simulink library "MIL_Test"  (Simulink 6.6)
undefined symbols (not defined in the file or in its folder): getdatatypespecs, slcm, StepSize
libraries: simulink x71, MIL_Test x6
(part 1 of 8)
settings Model: Creator=Justyna  LastModifiedBy=Justyna

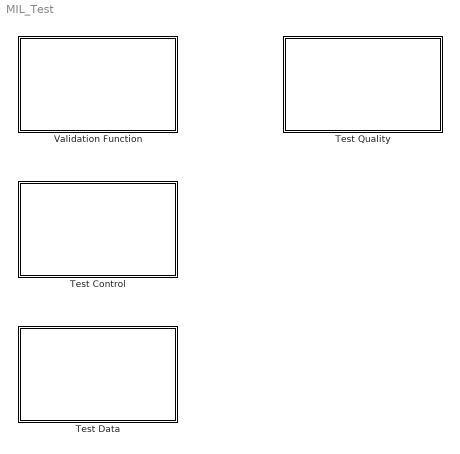
== system MIL_Test ==
  Test Control : Subsystem
  Test Data : Subsystem
  Test Quality : Subsystem
  Validation Function : Subsystem

== system MIL_Test/Test Control ==
  Test Control : Subsystem
  Test Control Architecture : Subsystem

== system MIL_Test/Test Data ==
  Feature generation : Subsystem
  Signal comparison : Subsystem
  Test Data Architecture : Subsystem

== system MIL_Test/Test Quality ==
  VFs Activation  Coverage : Subsystem  mask{req=9, So=on}
      mask prompts: req "Number of Evaluated Scenarios within Requirements"; So "Adjust to the present Eva Results"
      mask StyleString: popup(1|2|3|4|5|6|7|8|9|10|11|12|13|14|15|16|17|18|19|20),checkbox
      mask CallbackString: |Requirements_Coverage_callback(gcb,-1)

== system MIL_Test/Validation Function ==
  Assertions : MIL_Test/Validation Function/TODO/Assertions  SystemSampleTime=-1
  Feature extraction : Subsystem
  Preconditions : MIL_Test/Validation Function/TODO/Preconditions  SystemSampleTime=-1
  Signal comparison : Subsystem
  TODO : Subsystem
  Test Evaluation Architecture : Subsystem

== system MIL_Test/Test Control/Test Control ==

== system MIL_Test/Test Control/Test Control Architecture ==
  Connection Helpers : Subsystem
  Test Control  depending on Verdict : Subsystem  Orientation=left
  Test Control Conditions : Subsystem
  "independent  Test Control " : Stateflow chart  Orientation=left

== system MIL_Test/Test Data/Feature generation ==
  Generate  feature variants : Subsystem
  Generate  limited decrease : Subsystem  mask(Feature generation){X0=0.5, XF=0}
      mask prompts: X0 "Initial output:"; XF "Final output:"
      mask help: Output a decreasing ramp signal limited from bottom and top, starting at the specified time.
      mask Display:
      | plot([1:10],[4,4,4,4,4,1,1,1,1,1])
      | plot([1:10],[4,4,4,1,1,1,1,1,1,1])
      | plot([1:10],[4,1,1,1,1,1,1,1,1,1])
      | plot([1:10],[4,4,4,4,4,1,1,1,1,1])
      | plot([1:10],[4,4,4,4,4,4,4,1,1,1])
      | plot([1:10],[4,4,4,4,4,4,4,4,4,1])
      | plot([1:10],[4,4,4,4,4,4,4,4,4,4])
      | color('white');
      | plot([1:10],[1,1,1,1,1,1,1,1,1,1])
      | color('black');
      | plot([1,1.5],[1,1])
      | plot([2.5,3.5],[1,1])
      | plot([4.5,5.5],[1,1])
      | plot([6.5,7.5],[1,1])
      | plot([8.5,9.5],[1,1])
      | color('white');
      | plot([1,1.5],[4,4])
      | plot([2.5,3.5],[4,4])
      | plot([4.5,5.5],[4,4])
      | plot([6.5,7.5],[4,4])
      | plot([8.5,9.5],[4,4])
  Generate  limited decrease  with slope : Subsystem  mask(Feature generation){slope=-0.5, start=0, X0=100, XF=10, VectorParams1D=on}
      mask prompts: start "Start time:"; X0 "Initial output:"; XF "Final output:"; VectorParams1D "Interpret vector parameters as 1-D"
      mask help: Output a decreasing ramp signal limited from bottom and top, starting at the specified time.
      mask init:
      | blkName = gcb;
      | set_param([blkName '/Constant'], 'VectorParams1D',VectorParams1D);
      | set_param([blkName '/Constant1'], 'VectorParams1D',VectorParams1D);
      | set_param([blkName '/Step'], 'VectorParams1D',VectorParams1D);
      mask Display:
      | plot([1:10],[4,4,4,4,4,1,1,1,1,1])
      | plot([1:10],[4,4,4,4,4,4,4,4,4,4])
      | color('white');
      | plot([1:10],[1,1,1,1,1,1,1,1,1,1])
      | color('black');
      | plot([1,1.5],[1,1])
      | plot([2.5,3.5],[1,1])
      | plot([4.5,5.5],[1,1])
      | plot([6.5,7.5],[1,1])
      | plot([8.5,9.5],[1,1])
      | color('white');
      | plot([1,1.5],[4,4])
      | plot([2.5,3.5],[4,4])
      | plot([4.5,5.5],[4,4])
      | plot([6.5,7.5],[4,4])
      | plot([8.5,9.5],[4,4])
  Generate  limited increase : Subsystem  mask(Feature generation){X0=5, XF=14.5}
      mask prompts: X0 "Initial output:"; XF "Final output:"
      mask help: Output a ramp signal limited from bottom and top, starting at the specified time.
      mask Display:
      | plot([1:10],[1,1,1,1,1,4,4,4,4,4])
      | plot([1:10],[1,4,4,4,4,4,4,4,4,4])
      | plot([1:10],[1,1,1,4,4,4,4,4,4,4])
      | plot([1:10],[1,1,1,1,1,4,4,4,4,4])
      | plot([1:10],[1,1,1,1,1,1,1,4,4,4])
      | plot([1:10],[1,1,1,1,1,1,1,1,1,4])
      | plot([5:10],[1,1,1,1,1,1])
      | color('white');
      | plot([1:10],[4,4,4,4,4,4,4,4,4,4])
      | color('white');
      | plot([1,1.5],[1,1])
      | plot([2.5,3.5],[1,1])
      | plot([4.5,5.5],[1,1])
      | plot([6.5,7.5],[1,1])
      | plot([8.5,9.5],[1,1])
      | color('black');
      | plot([1,1.5],[4,4])
      | plot([2.5,3.5],[4,4])
      | plot([4.5,5.5],[4,4])
      | plot([6.5,7.5],[4,4])
      | plot([8.5,9.5],[4,4])
  Generate  limited increase  with slope : Subsystem  mask(Feature generation){slope=3.5, start=0, X0=10, XF=50, VectorParams1D=on}
      mask prompts: start "Start time:"; X0 "Initial output:"; XF "Final output:"; VectorParams1D "Interpret vector parameters as 1-D"
      mask help: Output a ramp signal limited from bottom and top, starting at the specified time.
      mask init: same as MIL_Test/Test Data/Feature generation/Generate  limited decrease  with slope
      mask Display:
      | plot([1:10],[1,1,1,1,1,4,4,4,4,4])
      | plot([5:10],[1,1,1,1,1,1])
      | color('white');
      | plot([1:10],[4,4,4,4,4,4,4,4,4,4])
      | color('white');
      | plot([1,1.5],[1,1])
      | plot([2.5,3.5],[1,1])
      | plot([4.5,5.5],[1,1])
      | plot([6.5,7.5],[1,1])
      | plot([8.5,9.5],[1,1])
      | color('black');
      | plot([1,1.5],[4,4])
      | plot([2.5,3.5],[4,4])
      | plot([4.5,5.5],[4,4])
      | plot([6.5,7.5],[4,4])
      | plot([8.5,9.5],[4,4])
  "Generate  local maximum  @ given time " : Subsystem  TreatAsAtomicUnit=on  mask(Feature generation){maxt=8, X0=10, XF=100}
      mask prompts: maxt "Time of Max:"; X0 "Lower Limit:"; XF "Upper Limit:"
      mask help: Generate local maximum
      mask Display:
      | plot([1:9],[1,1,1,1,4,1,1,1,1])
      | text(6,3,'@time')
  Generate  local maximum  with given slope : Subsystem  TreatAsAtomicUnit=on  mask(Feature generation){slope=7, start=5, maxt=8, X0=10, XF=100}
      mask prompts: start "Start Time of Feature:"; maxt "Time of Max:"; X0 "Lower Limit:"; XF "Upper Limit:"
      mask help: Generate local maximum
      mask Display:
      | plot([1:9],[1,1,1,1,4,1,1,1,1])
      | text(2,2,'slope')
      | text(6,3,'@time')
  Generate  local maximum = maxvalue  @ given time : Subsystem  TreatAsAtomicUnit=on  mask(Feature generation){maxv=50, maxt=5, X0=10}
      mask prompts: maxv "Value of Max:"; maxt "Time of Max:"; X0 "Lower Limit:"
      mask help: Generate local maximum = specified value
      mask Display:
      | plot([1:7],[1,1,4,1,1,1,1])
      | text(3.8,3.5,'max value')
      | text(4.1,2.5,'@time')
  Generate any step response  characteristics : Subsystem  mask(Feature generation){Param=0}
      mask prompts: Param "Mask Parameter 1:"
      mask help: Generate any step response characteristics
      mask Display:
      | plot([1:23],[-1,-1,-1,-1,0.3,1,1.5,1.7,1.5,0.7,0.4,0.6,1.1,1,0.6,0.7,0.7,0.7,0.7,0.7,0.7,0.7,0.7])
      | patch(0.17+[0.7 0.6 0.6 0.65 0.6 0.6 0.7],-0.043+[0.7 0.63 0.64 0.7 0.76 0.77 0.7],[0 0 0]);
  Generate complete step : Subsystem  mask(Complete step detection){Param=0}
      mask prompts: Param "Mask Parameter 1:"
      mask Display: plot([1,2,3,4,4.0001,6,7,7.0001,9,10],[1,1,1,1,4,4,4,2,2,2])
  Generate constant : Constant  Value=0  OutDataTypeMode=boolean
  Generate linear relation : Subsystem  mask(Feature generation){c=}
      mask prompts: c "Slope - c parameter:"
      mask help: Linear function y=cu
      mask Display:
      | plot([0:10],[0,1:10])
      | text(1,6.5,'y = c*u')
  Generate min to date : Subsystem  mask(Feature generation){low=-3, up=10}
      mask prompts: low "Min - Lower limit:"; up "Max - Upper limit:"
      mask help: Generate any characteristics
      mask Display:
      | port_label('output',1,'Min to date');
      | patch(0.05+[0.25 0.25 0.8 0.8 0.26 0.26],[0.95 0.65 0.65 0.66 0.66 0.95],[0 0 0]);
      | patch(0.033+[0.27 0.22 0.23 0.27 0.31 0.32 0.27],0.02+[0.95 0.85 0.85 0.89 0.85 0.85 0.95],[0 0 0]);
      | patch(0.27+[0.7 0.6 0.6 0.65 0.6 0.6 0.7],-0.043+[0.7 0.63 0.64 0.7 0.76 0.77 0.7],[0 0 0]);
      | patch(0.05+[0.25 0.25 0.25 0.5 0.26 0.26],0.05+[0.65 0.65 0.65 0.66 0.66 0.95],[0 0 0]);
  Generate peaks : Subsystem  TreatAsAtomicUnit=on  mask(Feature generation){Sens=0.910, freq=1}
      mask prompts: Sens "Peak value:"; freq "Peaks frequency:"
      mask help: Generate a peak in a signal. The peak might be positive or negative. The user-defined parameter define the minimal peak size and frequency of peak occurence.
      mask CallbackString:
      | if str2double(get_param(gcb,'Sens')) <= 0
      |     error(['Sensibility value (' get_param(gcb,'Sens') ') out of range. Please give a value greater than zero.']);
      | end|
      mask Display:
      | plot([1:10],[1,1,2,0,2,1,2,0,1,1])
      | patch(0.17+[0.7 0.6 0.6 0.65 0.6 0.6 0.7],-0.043+[0.7 0.63 0.64 0.7 0.76 0.77 0.7],[0 0 0]);
  Generate signal  crossing a given value  @ given time : Subsystem  TreatAsAtomicUnit=on  mask(Feature generation){val=20, time=5, up=50, low=10}
      mask prompts: val "Value of signal:"; time "Time of event:"; up "Upper Limit:"; low "Lower Limit:"
      mask help: Generate signal crossing a given value @ given time
      mask Display:
      | port_label('output',1,'Feature');
      | patch(0.05+[0.25 0.25 0.8 0.8 0.26 0.26],[0.95 0.65 0.65 0.66 0.66 0.95],[0 0 0]);
      | patch(0.033+[0.27 0.22 0.23 0.27 0.31 0.32 0.27],0.02+[0.95 0.85 0.85 0.89 0.85 0.85 0.95],[0 0 0]);
      | patch(0.27+[0.7 0.6 0.6 0.65 0.6 0.6 0.7],-0.043+[0.7 0.63 0.64 0.7 0.76 0.77 0.7],[0 0 0]);
      | patch(0.16+[0.25 0.25 0.8 0.8 0.26 0.26],[0.8 0.65 0.65 0.66 0.66 0.8],[0 0 0]);
      | patch(0.05+[0.25 0.25 0.25 0.4 0.26 0.26],0.05+[0.65 0.65 0.65 0.66 0.66 0.95],[0 0 0]);
  Generate signal which  starts to be constant @ time : Subsystem  TreatAsAtomicUnit=on  mask(Feature generation){ST=10, const=2}
      mask prompts: ST "Start time of constant signal:"; const "Value of constant"
      mask help: Generate sinus signal till the desired point of time where it is constant
      mask Display: plot([1:9],[1,3,2,4,2,2,2,2,2])
  Generate step : Step  After=StepSize  SampleTime=0

== system MIL_Test/Test Data/Signal comparison ==
  Bound Precond : Subsystem  mask(Bound){cm=>=}
      mask prompts: cm "Comparison method:"
      mask help:
      | Compare a signal with a reference using the specified comparison method.
      |
      | For '==' or '~=' use "Range - Gap"
      mask init:
      | bp = get_param(gcbh,'Parent');
      | bn = get_param(gcbh,'Name');
      | set_param([bp '/' bn '/RelOp'],'Operator',get_param(gcbh,'cm'));
      mask StyleString: popup(>|>=|<=|<)
      mask Display:
      | port_label('output', 1, 'A');
      | port_label('input', 1, 'Sig');
      | port_label('input', 2, 'Ref');
      | text(0.05,0.5,get_param(get_param([get_param(gcb,'Parent') '/' get_param(gcb,'Name') '/RelOp'],'handle'),'Operator'));
  Range - Gap Absolute tolerance Precond : Subsystem  mask(Range - Gap Absolute Tolerance){GorR=Range, AbsoluteTolerance=100}
      mask prompts: GorR "Use range or gap"; AbsoluteTolerance "Absolute Tolerance"
      mask help: Check that a signal stays inside a range or outside a gap around a reference signal. Specify the range or the gap absolute to the reference signal.
      mask init:
      | if max(get_param(gcb,'GorR') == ' ') % Gap
      |     helpVariable1 = '~=';
      | else % Range
      |     helpVariable1 = '==';
      | end
      | set_param([gcb '/Relational Operator'],'Operator',helpVariable1);
      mask StyleString: popup(Range|Gap  ),edit
      mask Display:
      | port_label('output',1,'A');
      | port_label('input',1,'Sig');
      | port_label('input',2,'Ref');
      | text(0.40,0.53,'+');
      | text(0.415,0.46,'-');
      | text(0.5,0.5,num2str(AbsoluteTolerance));
      | text(0.05,0.5,helpVariable1);
  Range - Gap Relative tolerance Precond : Subsystem  mask(Range - Gap Relative Tolerance){GorR=Range, RelativeTolerance=0.0001}
      mask prompts: GorR "Use range or gap"; RelativeTolerance "Relative Tolerance in Percent"
      mask help: Check that a signal stays inside a range or outside a gap around a reference signal. Specify the range or the gap relative to the reference signal.
      mask init:
      | if max(get_param(gcb,'GorR') == ' ') % Gap
      |     helpVariable1 = '>=';
      |     helpVariable2 = '~=';
      | else % Range
      |     helpVariable1 = '<=';
      |     helpVariable2 = '==';
      | end
      | set_param([get_param(gcb,'Parent') '/' get_param(gcb,'Name') '/Relational Operator'],'Operator',helpVariable1);
      | clear helpVariable1;
      mask StyleString: popup(Range|Gap  ),edit
      mask Display:
      | port_label('output',1,'A');
      | port_label('input',1,'Sig');
      | port_label('input',2,'Ref');
      | text(0.35,0.5,[num2str(RelativeTolerance) '%']);
      | text(0.05,0.5,helpVariable2);
  Range - Gap Tolerance range Precond : Subsystem  mask(Range - Gap Tolerance range){GorR=Range}
      mask prompts: GorR "Use range or gap"
      mask help: Check that a signal stays inside a dynamically specified value range.
      mask init:
      | if max(get_param(gcb,'GorR') == ' ') % Gap
      |     helpVariable1 = '<=';
      | else % Range
      |     helpVariable1 = '>=';
      | end
      | set_param([gcb '/Relational Operator'],'Operator',helpVariable1);
      mask StyleString: popup(Range|Gap  )
      mask Display:
      | port_label('output',1,'A');
      | port_label('input',1,'Sig');
      | port_label('input',2,'Lower Bound');
      | port_label('input',3,'Upper Bound');
      | patch(0.05+[0.3 0.7 0.7 0.3],-0.05+[0.8 0.8 0.9 0.9],[1 1 1]*double(not(max(get_param(gcb,'GorR') == ' '))));
      | patch(0.05+[0.3 0.7 0.7 0.3],-0.05+[0.9 0.9 0.95 0.95],[1 1 1]*double(max(get_param(gcb,'GorR') == ' ')));
      | patch(0.05+[0.3 0.7 0.7 0.3],-0.05+[0.75 0.75 0.8 0.8],[1 1 1]*double(max(get_param(gcb,'GorR') == ' ')));
      | patch(0.05+[0.25 0.25 0.8 0.8 0.26 0.26],[0.95 0.65 0.65 0.66 0.66 0.95],[0 0 0]);
      | patch(0.033+[0.27 0.22 0.23 0.27 0.31 0.32 0.27],0.02+[0.95 0.85 0.85 0.89 0.85 0.85 0.95],[0 0 0]);
      | patch(0.17+[0.7 0.6 0.6 0.65 0.6 0.6 0.7],-0.043+[0.7 0.63 0.64 0.7 0.76 0.77 0.7],[0 0 0]);

== system MIL_Test/Test Data/Test Data Architecture ==
  <Test data generator> : Subsystem  mask{No=1, So=1, T=off}
      mask prompts: No "Number of Requirements"; So "Number of Signals"; T "Do you want to shut off the mask"
      mask StyleString: popup(1|2|3|4|5|6|7|8|9|10|11|12|13|14|15|16|17|18|19|20),popup(1|2|3|4|5|6|7|8|9|10|11|12|13|14|15|16|17|18|19|20),checkbox
      mask CallbackString: Test_D_Gen(gcb);|Test_D_Gen_S(gcb,-1);|shut_mask(gcb);

== system MIL_Test/Test Quality/VFs Activation  Coverage ==
  VF Bus : Inport
  Bus Selector : BusSelector  OutputSignals=Local Verdicts.signal1.signal1.signal1.Local verdict,Local Verdicts.signal1.signal1.signal2.Local verdict
  Data Type Conversion : DataTypeConversion
  Divide : Product  Inputs=*/  OutScaling=2^-10
  Max to date : Subsystem  TreatAsAtomicUnit=on
  Max to date1 : Subsystem  TreatAsAtomicUnit=on
  Requirements Coverage : Display
  Sum : Sum  Inputs=|++
  nb of scenarios : Constant  Value=req
  percentage : Gain  Gain=100
  verdict is  not none : simulink/Logic and Bit Operations/Compare To Constant  SystemSampleTime=-1  relop=~=  const=2  LogicOutDataTypeMode=uint8  ZeroCross=off
  verdict is  not none1 : simulink/Logic and Bit Operations/Compare To Constant  SystemSampleTime=-1  relop=~=  const=2  LogicOutDataTypeMode=uint8  ZeroCross=off
  RC : Outport
  wires:
  VF Bus/1 -> Bus Selector/1
  Bus Selector/1 -> verdict is  not none/1  "<Local verdict>"
  Bus Selector/2 -> verdict is  not none1/1  "<Local verdict>"
  Sum/1 -> Requirements Coverage/1, Data Type Conversion/1
  percentage/1 -> RC/1
  Data Type Conversion/1 -> Divide/1
  verdict is  not none/1 -> Max to date/1(Signal)
  verdict is  not none1/1 -> Max to date1/1(Signal)
  Divide/1 -> percentage/1
  nb of scenarios/1 -> Divide/2
  Max to date/1(Max) -> Sum/1
  Max to date1/1(Max) -> Sum/2

== system MIL_Test/Validation Function/Feature extraction ==
  Complete step detection : Subsystem  mask(Complete step detection){Param=0}
      mask prompts: Param "Mask Parameter 1:"
  Detect constant : Subsystem  TreatAsAtomicUnit=on  mask(Feature extraction block){RT=1}
      mask prompts: RT "Relative tolerance in %"
      mask help: Detect if the signal value is constant (using the last two signal values) allowing for a user-defined relative deviation
      mask CallbackString:
      | if or( (str2double(get_param(gcb,'RT')) < 0), (str2double(get_param(gcb,'RT')) > 100))
      |     error(['Relative tolerance value (' get_param(gcb,'RT') ') out of range. Please give a value between 0 and 100.']);
      | else
      |     set_param([gcb '/Relative tolerance/Relative Tolerance'],'Value',get_param(gcb,'RT'));
      | end
  Detect decrease : Subsystem  TreatAsAtomicUnit=on  mask(Detect increase){Param=0}
      mask prompts: Param "Mask Parameter 1:"
  Detect increase : Subsystem  TreatAsAtomicUnit=on  mask(Detect increase){Param=0}
      mask prompts: Param "Mask Parameter 1:"
  Linear relation : Subsystem  TreatAsAtomicUnit=on  mask(Feature extraction block){c=5, RT=0.1}
      mask prompts: c "Linearity constant"; RT "Relative tolerance in %"
      mask help:
      | Detect if the signals u and y are linearly dependent. The parameter c represents the linear constant.
      |
      | Deviations of the linear law are permitted within user-defined limits (Parameter relative tolerance).
      mask CallbackString:
      | set_param([gcb '/c'],'Value',get_param(gcb,'c'));|if or( (str2double(get_param(gcb,'RT')) < 0), (str2double(get_param(gcb,'RT')) > 100))
      |     error(['Relative tolerance value (' get_param(gcb,'RT') ') out of range. Please give a value between 0 and 100.']);
      | else
      |     set_param([gcb '/Relative tolerance/Relative Tolerance'],'Value',get_param(gcb,'RT'));
      | end
  Local maximum : Subsystem  TreatAsAtomicUnit=on  mask(Local maximum){Param=0}
      mask prompts: Param "Mask Parameter 1:"
  Min to date : Subsystem  TreatAsAtomicUnit=on  mask(Min to date){Param=0}
      mask prompts: Param "Mask Parameter 1:"
  Moving average : Subsystem  TreatAsAtomicUnit=on  mask(Moving average){Param=0}
      mask prompts: Param "Mask Parameter 1:"
  Peak detection : Subsystem  TreatAsAtomicUnit=on  mask(Feature extraction block){Sens=0.198}
      mask prompts: Sens "Detection sensibility"
      mask help: Detect a peak in a signal. The peak might be positive or negative. The user-defined parameter define the minimal peak size for detection.
      mask CallbackString:
      | if str2double(get_param(gcb,'Sens')) <= 0
      |     error(['Sensibility value (' get_param(gcb,'Sens') ') out of range. Please give a value greater than zero.']);
      | else
      |     set_param([gcb '/Sensibility1'],'Value',get_param(gcb,'Sens'));
      |     set_param([gcb '/Sensibility2'],'Value',get_param(gcb,'Sens'));
      | end
  Signal value @ maximum : Subsystem  TreatAsAtomicUnit=on  mask(Signal value @ maximum){Param=0}
      mask prompts: Param "Mask Parameter 1:"
  Step detection : Subsystem  TreatAsAtomicUnit=on  mask(Feature extraction block){StepSize=1}
      mask prompts: StepSize "Minimum step size"
      mask help: Detect a step in the signal. The minimum step size is defined by the user.
      mask CallbackString:
      | if str2double(get_param(gcb,'StepSize')) <= 0
      |     error(['Minimum step size (' get_param(gcb,'StepSize') ') out of range. Please give a value greater than zero.']);
      | else
      |     set_param([gcb '/Min step size'],'Value',get_param(gcb,'StepSize'));
      | end
  Step response characteristics : Subsystem  mask(Step response characteristics){Param=0}
      mask prompts: Param "Mask Parameter 1:"
  Time @ sig = x : Subsystem  TreatAsAtomicUnit=on  mask(Feature extraction block){x=5, RT=1}
      mask prompts: x "Trigger value"; RT "Relative tolerance in %"
      mask help: Trigger the actual time when the input signal has a certain value (use a tolerance range).
      mask CallbackString:
      | if or( (str2double(get_param(gcb,'RT')) < 0), (str2double(get_param(gcb,'RT')) > 100))
      |     error(['Relative tolerance value (' get_param(gcb,'RT') ') out of range. Please give a value between 0 and 100.']);
      | else
      |     set_param([gcb '/Relative tolerance/Relative Tolerance'],'Value',get_param(gcb,'RT'));
      |     set_param([gcb '/Trigger Value'],'Value',get_param(gcb,'x'));
      | end|if or( (str2double(get_param(gcb,'RT')) < 0), (str2double(get_param(gcb,'RT')) > 100))
      |     error(['Relative tolerance value (' get_param(gcb,'RT') ') out of range. Please give a value between 0 and 100.']);
      | else
      |     set_param([gcb '/Relative tolerance/Relative Tolerance'],'Value',get_param(gcb,'RT'));
      |     set_param([gcb '/Trigger Value'],'Value',get_param(gcb,'x'));
      | end
  Time since signal constant : Subsystem  TreatAsAtomicUnit=on  mask(Feature extraction block){RT=1}
      mask prompts: RT "Relative tolerance in %"
      mask help: Detect if the signal value is constant (using the last two signal values) allowing for a user-defined relative deviation
      mask CallbackString:
      | if or( (str2double(get_param(gcb,'RT')) < 0), (str2double(get_param(gcb,'RT')) > 100))
      |     error(['Relative tolerance value (' get_param(gcb,'RT') ') out of range. Please give a value between 0 and 100.']);
      | else
      |     set_param([gcb '/Detect constant/Relative tolerance/Relative Tolerance'],'Value',get_param(gcb,'RT'));
      | end

== system MIL_Test/Validation Function/Signal comparison ==
  Bound Ass : Subsystem  mask(Bound){cm=<=, Lower=1, Upper=0, Ass=[1 2], Pre=[1 2], Req=[1 2]}
      mask prompts: cm "Comparison method:"; Upper "Mask Parameter 3:"; Req "Mask Parameter 6:"
      mask help:
      | Compare a signal with a reference using the specified comparison method.
      |
      | Output verdict V and lower (LL) and upper (UL) limits for reporting.
      |
      | For '==' or '~=' use "Range - Gap"
      mask init:
      | set_param([get_param(gcb,'Parent') '/' get_param(gcb,'Name') '/Relational Operator'],'Operator',get_param(gcb,'cm'));
      | set_param(gcb,'Upper',num2str(uint8(max(get_param([get_param(gcb,'Parent') '/' get_param(gcb,'Name') '/Relational Operator'],'Operator') == '>'))));
      | set_param(gcb,'Lower',num2str(uint8(max(get_param([get_param(gcb,'Parent') '/' get_param(gcb,'Name') '/Relational Operator'],'Operator') == '<'))));
      | set_param(gcb, ...
      |           'Ass', ...
      |           ['[1 2]']);
      | set_param(gcb, ...
      |           'Pre', ...
      |           ['[1 2]']); 
      | set_param(gcb, ...
      |           'Req', ...
      |           ['[1 2]']);
      mask StyleString: popup(>|>=|<=|<),edit,edit,edit,edit,edit
      mask Display:
      | port_label('output', 1, ['V']);
      | port_label('input', 1, 'Sig');
      | port_label('input', 2, 'Ref');
      | text(0.05,0.5,get_param(get_param([get_param(gcb,'Parent') '/' get_param(gcb,'Name') '/Relational Operator'],'handle'),'Operator'));
  Bound Precond : Subsystem  mask(Bound){cm=>=}
      mask prompts: cm "Comparison method:"
      mask help:
      | Compare a signal with a reference using the specified comparison method.
      |
      | For '==' or '~=' use "Range - Gap"
      mask init:
      | bp = get_param(gcbh,'Parent');
      | bn = get_param(gcbh,'Name');
      | set_param([bp '/' bn '/RelOp'],'Operator',get_param(gcbh,'cm'));
      mask StyleString: popup(>|>=|<=|<)
      mask Display:
      | port_label('output', 1, 'A');
      | port_label('input', 1, 'Sig');
      | port_label('input', 2, 'Ref');
      | text(0.05,0.5,get_param(get_param([get_param(gcb,'Parent') '/' get_param(gcb,'Name') '/RelOp'],'handle'),'Operator'));
  Range - Gap Absolute tolerance Ass : Subsystem  mask(Range - Gap Absolute Tolerance){GorR=Range, AbsoluteTolerance=100}
      mask prompts: GorR "Use range or gap"; AbsoluteTolerance "Absolute Tolerance"
      mask help: Check that a signal stays inside a range or outside a gap around a reference signal. Specify the range or the gap absolute to the reference signal.
      mask init:
      | if max(get_param(gcb,'GorR') == ' ') % Gap
      |     helpVariable1 = '~=';
      | else % Range
      |     helpVariable1 = '==';
      | end
      | set_param([gcb '/Relational Operator'],'Operator',helpVariable1);
      mask StyleString: popup(Range|Gap  ),edit
      mask Display:
      | port_label('output',1,'V');
      | port_label('input',1,'Sig');
      | port_label('input',2,'Ref');
      | text(0.40,0.53,'+');
      | text(0.415,0.46,'-');
      | text(0.5,0.5,num2str(AbsoluteTolerance));
      | text(0.05,0.5,helpVariable1);
  Range - Gap Absolute tolerance Precond : Subsystem  mask(Range - Gap Absolute Tolerance){GorR=Range, AbsoluteTolerance=100}
      mask prompts: GorR "Use range or gap"; AbsoluteTolerance "Absolute Tolerance"
      mask help: Check that a signal stays inside a range or outside a gap around a reference signal. Specify the range or the gap absolute to the reference signal.
      mask init:
      | if max(get_param(gcb,'GorR') == ' ') % Gap
      |     helpVariable1 = '~=';
      | else % Range
      |     helpVariable1 = '==';
      | end
      | set_param([gcb '/Relational Operator'],'Operator',helpVariable1);
      mask StyleString: popup(Range|Gap  ),edit
      mask Display:
      | port_label('output',1,'A');
      | port_label('input',1,'Sig');
      | port_label('input',2,'Ref');
      | text(0.40,0.53,'+');
      | text(0.415,0.46,'-');
      | text(0.5,0.5,num2str(AbsoluteTolerance));
      | text(0.05,0.5,helpVariable1);
  Range - Gap Relative tolerance Ass : Subsystem  mask(Range - Gap Relative Tolerance){GorR=Range, RelativeTolerance=0.0001}
      mask prompts: GorR "Use range or gap"; RelativeTolerance "Relative Tolerance in Percent"
      mask help: Check that a signal stays inside a range or outside a gap around a reference signal. Specify the range or the gap relative to the reference signal.
      mask init: same as MIL_Test/Test Data/Signal comparison/Range - Gap Relative tolerance Precond
      mask StyleString: popup(Range|Gap  ),edit
      mask Display:
      | port_label('output',1,'V');
      | port_label('input',1,'Sig');
      | port_label('input',2,'Ref');
      | text(0.35,0.5,[num2str(RelativeTolerance) '%']);
      | text(0.05,0.5,helpVariable2);
  Range - Gap Relative tolerance Precond : Subsystem  mask(Range - Gap Relative Tolerance){GorR=Range, RelativeTolerance=0.0001}
      mask prompts: GorR "Use range or gap"; RelativeTolerance "Relative Tolerance in Percent"
      mask help: Check that a signal stays inside a range or outside a gap around a reference signal. Specify the range or the gap relative to the reference signal.
      mask init: same as MIL_Test/Test Data/Signal comparison/Range - Gap Relative tolerance Precond
      mask StyleString: popup(Range|Gap  ),edit
      mask Display:
      | port_label('output',1,'A');
      | port_label('input',1,'Sig');
      | port_label('input',2,'Ref');
      | text(0.35,0.5,[num2str(RelativeTolerance) '%']);
      | text(0.05,0.5,helpVariable2);
  Range - Gap Tolerance range Ass : Subsystem  mask(Range - Gap Tolerance range){GorR=Range}
      mask prompts: GorR "Use range or gap"
      mask help: Check that a signal stays inside a dynamically specified value range.
      mask init:
      | if max(get_param(gcb,'GorR') == ' ') % Gap
      |     helpVariable1 = '<=';
      | else % Range
      |     helpVariable1 = '>=';
      | end
      | set_param([gcb '/Relational Operator'],'Operator',helpVariable1);
      mask StyleString: popup(Range|Gap  )
      mask Display:
      | port_label('output',1,'V');
      | port_label('input',1,'Sig');
      | port_label('input',2,'Lower Bound');
      | port_label('input',3,'Upper Bound');
      | patch(0.05+[0.3 0.7 0.7 0.3],-0.05+[0.8 0.8 0.9 0.9],[1 1 1]*double(not(max(get_param(gcb,'GorR') == ' '))));
      | patch(0.05+[0.3 0.7 0.7 0.3],-0.05+[0.9 0.9 0.95 0.95],[1 1 1]*double(max(get_param(gcb,'GorR') == ' ')));
      | patch(0.05+[0.3 0.7 0.7 0.3],-0.05+[0.75 0.75 0.8 0.8],[1 1 1]*double(max(get_param(gcb,'GorR') == ' ')));
      | patch(0.05+[0.25 0.25 0.8 0.8 0.26 0.26],[0.95 0.65 0.65 0.66 0.66 0.95],[0 0 0]);
      | patch(0.033+[0.27 0.22 0.23 0.27 0.31 0.32 0.27],0.02+[0.95 0.85 0.85 0.89 0.85 0.85 0.95],[0 0 0]);
      | patch(0.17+[0.7 0.6 0.6 0.65 0.6 0.6 0.7],-0.043+[0.7 0.63 0.64 0.7 0.76 0.77 0.7],[0 0 0]);
  Range - Gap Tolerance range Precond : Subsystem  mask(Range - Gap Tolerance range){GorR=Range}
      mask prompts: GorR "Use range or gap"
      mask help: Check that a signal stays inside a dynamically specified value range.
      mask init:
      | if max(get_param(gcb,'GorR') == ' ') % Gap
      |     helpVariable1 = '<=';
      | else % Range
      |     helpVariable1 = '>=';
      | end
      | set_param([gcb '/Relational Operator'],'Operator',helpVariable1);
      mask StyleString: popup(Range|Gap  )
      mask Display:
      | port_label('output',1,'A');
      | port_label('input',1,'Sig');
      | port_label('input',2,'Lower Bound');
      | port_label('input',3,'Upper Bound');
      | patch(0.05+[0.3 0.7 0.7 0.3],-0.05+[0.8 0.8 0.9 0.9],[1 1 1]*double(not(max(get_param(gcb,'GorR') == ' '))));
      | patch(0.05+[0.3 0.7 0.7 0.3],-0.05+[0.9 0.9 0.95 0.95],[1 1 1]*double(max(get_param(gcb,'GorR') == ' ')));
      | patch(0.05+[0.3 0.7 0.7 0.3],-0.05+[0.75 0.75 0.8 0.8],[1 1 1]*double(max(get_param(gcb,'GorR') == ' ')));
      | patch(0.05+[0.25 0.25 0.8 0.8 0.26 0.26],[0.95 0.65 0.65 0.66 0.66 0.95],[0 0 0]);
      | patch(0.033+[0.27 0.22 0.23 0.27 0.31 0.32 0.27],0.02+[0.95 0.85 0.85 0.89 0.85 0.85 0.95],[0 0 0]);
      | patch(0.17+[0.7 0.6 0.6 0.65 0.6 0.6 0.7],-0.043+[0.7 0.63 0.64 0.7 0.76 0.77 0.7],[0 0 0]);

== system MIL_Test/Validation Function/TODO ==
  <system name> : Subsystem  Description=Test evaluation system template. Create a new test evaluation system from this template.
  Assertion:  SpeedMaintenance : Stateflow chart
  Assertions : Subsystem
  Bus Creator : BusCreator  Inputs=1
  Model Info : Subsystem  LoadFcn=slcm LoadBlock;  InitFcn=slcm('UpdateAllCMBlocksInThisModelInit')  mask(CMBlock){InitialSaveTempField=, InitialBlockCM=None, BlockCM=None, Frame=on, SaveTempField=, DisplayStringWithTags=|, MaskDisplayString=TI  - Trigger Independent\nTD - Trigger Dependent, HorizontalTextAlignment=Center, LeftAlignmentValue=0.5, SourceBlockDiagram=MIL_Test, TagMaxNumber=20, CMTag1=, CMTag2=, CMTag3=, CMTag4=, CMTag5=, CMTag6=, CMTag7=, CMTag8=, CMTag9=, CMTag10=, CMTag11=, CMTag12=, CMTag13=, CMTag14=, CMTag15=, CMTag16=, CMTag17=, CMTag18=, CMTag19=, CMTag20=}
      mask DisplayStringWithTags=|
      | TI  - Trigger Independent
      | TD - Trigger Dependent
      mask help: This block allows revision control information to be displayed within the model.
      settings: CopyFcn=slcm CopyBlock;  DeleteFcn=slcm Cancel;  PostSaveFcn=slcm('UpdateAllCMBlocksInThisModel')  NameChangeFcn=slcm Rename;  OpenFcn=slcm
      mask Display: text(str2num(LeftAlignmentValue), 0.5, MaskDisplayString, 'HorizontalAlignment', HorizontalTextAlignment)
  Preconditions : Subsystem
  TD determinate (TD D) : Subsystem
  TD immediate (TD I) : Subsystem
  TD indeterminate : Subsystem
  "TD indeterminate, limited (TD IL)" : Subsystem
  TI determinate (TI D) : Subsystem
  TI immediate (TI I) : Subsystem
  User-defined target:  Active_30 : Stateflow chart
  Validation FunctionsTemplate : Subsystem  mask{No=2}
      mask prompts: No "Number of Requirements"
      mask StyleString: popup(1|2|3|4|5|6|7|8|9|10|11|12|13|14|15|16|17|18|19|20)
      mask CallbackString: VFs_callback(gcb);
  wires:
  Bus Creator/1 -> <system name>/1(InOut Bus)  "InOut Bus"

== system MIL_Test/Validation Function/Test Evaluation Architecture ==
  <system name> : Subsystem  Description=Test evaluation system template. Create a new test evaluation system from this template.  mask{No=1, T=off}
      mask prompts: No "Number of Requirements"; T "Shut off the mask"
      mask StyleString: popup(1|2|3|4|5|6|7|8|9|10|11|12|13|14|15|16|17|18|19|20),checkbox
      mask CallbackString: system_name2(gcb);|shut_mask(gcb);
  Alternative : Subsystem

== system MIL_Test/Test Control/Test Control Architecture/Connection Helpers ==
  TestControl for  TestCases Sequencing : Subsystem  Orientation=left  mask(Specify the Input Signals Influencing Test Control){No=0, NoDuring=0, NoAtTime=0}
      mask prompts: No "Check the Signal Overall Value at the End of Simulation:"; NoDuring "Check the Signal Values during a given period of Time:"; NoAtTime "Check the Signal Value at a given Time:"
      mask help:
      | Specify the Input Signals Influencing Test Control. They can be the following:
      | - IF Signal@SimStopTime for TC = value
      | - IF signal @[timeUp, timeDown] for TC = value
      | - IF signal@time for TC = value
      mask StyleString: popup(0|1|2|3|4|5|6|7|8|9|10|11|12|13|14),popup(0|1|2|3|4|5|6|7|8|9|10|11|12|13|14),popup(0|1|2|3|4|5|6|7|8|9|10|11|12|13|14)
      mask CallbackString:
      | TCtrlStopTime_callback(gcb);
      | |TCtrlDuring_callback(gcb);
      | |TCtrlAtTime_callback(gcb);
  TestControl for  TestCases Sequencing NoMask : Subsystem  Orientation=left
  TestControl for  TestCases SequencingTemplate : Subsystem  Orientation=left  mask(Specify the Input Signals Influencing Test Control){No=0, NoDuring=0, NoAtTime=0}
      mask prompts: No "Check the Signal Overall Value at the End of Simulation:"; NoDuring "Check the Signal Values during a given period of Time:"; NoAtTime "Check the Signal Value at a given Time:"
      mask help:
      | Specify the Input Signals Influencing Test Control. They can be the following:
      | - IF Signal@SimStopTime for TC = value
      | - IF signal @[timeUp, timeDown] for TC = value
      | - IF signal@time for TC = value
      mask StyleString: popup(0|1|2|3|4|5|6|7|8|9|10|11|12|13|14),popup(0|1|2|3|4|5|6|7|8|9|10|11|12|13|14),popup(0|1|2|3|4|5|6|7|8|9|10|11|12|13|14)
      mask CallbackString:
      | TCtrlStopTime_callback(gcb);
      | |TCtrlDuring_callback(gcb);
      | |TCtrlAtTime_callback(gcb);

== system MIL_Test/Test Control/Test Control Architecture/Test Control  depending on Verdict ==
  Out Bus : Inport
  Bus Selector : BusSelector  OutputSignals=signal2.signal1.signal1.signal1.signal1.Local verdict
  Counter : Subsystem
  Memory : Memory
  OR : Logic  Operator=OR  Inputs=3  AllPortsSameDT=off  OutDataTypeMode=Boolean
  Switch : Switch  Criteria=u2 > Threshold
  error : simulink/Logic and Bit Operations/Compare To Constant  SystemSampleTime=-1  relop===  const=-1  LogicOutDataTypeMode=uint8  ZeroCross=off
  fail : simulink/Logic and Bit Operations/Compare To Constant  SystemSampleTime=-1  relop===  const=0  LogicOutDataTypeMode=uint8  ZeroCross=off
  pass : simulink/Logic and Bit Operations/Compare To Constant  SystemSampleTime=-1  relop===  const=1  LogicOutDataTypeMode=uint8  ZeroCross=off
  test case 1 : Constant
  test case 2 : Constant  Value=2
  Test Control : Outport
  wires:
  OR/1 -> Counter/1(In1), Counter/Trigger
  test case 1/1 -> Switch/3
  Out Bus/1 -> Bus Selector/1
  Switch/1 -> Test Control/1
  test case 2/1 -> Switch/1
  Counter/1(Out1) -> Switch/2
  Bus Selector/1 -> Memory/1  "<Local verdict>"
  pass/1 -> OR/1
  fail/1 -> OR/2
  error/1 -> OR/3
  Memory/1 -> pass/1, error/1, fail/1

== system MIL_Test/Test Control/Test Control Architecture/Test Control Conditions ==
  IF Signal@SimStopTime for TC = value1 : Subsystem  mask(Check if Incoming Signal has an Expected Value @ Simulation Stop Time){currentStopTime=on, condition=0}
      mask prompts: currentStopTime "Check @ End of Simulation"; condition "Signal should equal to"
      mask help:
      | The Subsystem checks if the incoming signal (i.e. Overall Verdict, single Requirement Local Verdict, or SUT Outputs) has an expected value at the end of simulation of a previously specified testcase.
      | ____________________________________________________________________
      | 'Check @ End of Simulation' gets the simulation stop time from the window in Simulink.
      | 'Signal should equal to:' is used for giving the condition for the value of signal (i.e.):
      | 2 = none
      | 1 = pass
      | 0 = fail
      | X = anyNumber
      | The subsystem outputs 1 if the condition is fullfilled.
      mask init:
      | % p=get_param(gcb, 'PortHandles');
      | % l=get_param(p.Inport, 'Line'); 
      | % Inp=get_param(p.Inport, 'Name');
      | % set_param(Inp, 'Name', get_param(l, 'Name'));
      mask CallbackString:
      | block = gcb;
      | TCtblock = get_param(get_param(block, 'Parent'), 'Parent');
      | currentStopTime = get_param(TCtblock, 'StopTime');|
  "IF signal @[timeUp, timeDown] for TC = value1" : Subsystem  mask(Check if Incoming Signal has an Expected Value in the given Period of Time){timeDown=11, timeUp=155, condition=1}
      mask prompts: timeDown "Check @ Time from:"; timeUp "Check @ Time till:"; condition "Signal should equal to:"
      mask help:
      | The Subsystem checks if the incoming signal (i.e. Overall Verdict, single Requirement Local Verdict, or SUT Outputs) has an expected value in the given period of time of a previously specified testcase.
      | ____________________________________________________________________
      | 'Check @ Time from:' means the time where the check should begin.
      | 'Check @ Time till:' means the time where the check should end.
      | Constraint: TimeUp > TimeDown.
      | 'Signal should equal to:' is used for giving the condition for the value of signal (i.e.):
      | 2 = none
      | 1 = pass
      | 0 = fail
      | X = anyNumber
      | The subsystem outputs 1 if the condition is fullfilled.
      mask init:
      | % p=get_param(gcb, 'PortHandles');
      | % l=get_param(p.Inport, 'Line'); 
      | % Inp=get_param(p.Inport, 'Name');
      | % set_param(Inp, 'Name', get_param(l, 'Name'));
      mask CallbackString: timeDown = str2double(get_param(gcb,'timeDown'));|timeUp = str2double(get_param(gcb,'timeUp'));|
  IF signal@time for TC = value1 : Subsystem  mask(Check if Incoming Signal has an Expected Value @ given Time){time=22, condition=1}
      mask prompts: time "Check @ Time t"; condition "Signal should equal to"
      mask help:
      | The Subsystem checks if the incoming signal (i.e. Overall Verdict, single Requirement Local Verdict, or SUT Outputs) has an expected value at given time of a previously specified testcase.
      | ____________________________________________________________________
      | 'Check @ Time t' means the time point when the condition should be checked.
      | 'Signal should equal to:' is used for giving the condition for the value of signal (i.e.):
      | 2 = none
      | 1 = pass
      | 0 = fail
      | X = anyNumber
      | The subsystem outputs 1 if the condition is fullfilled.
      mask CallbackString: time = str2double(get_param(gcb,'time'));|
  IF signal@time1 : Subsystem  mask(Check if Incoming Signal has an Expected Value @ Simulation Stop Time){currentStopTime=on, condition=0}
      mask prompts: currentStopTime "Check @ End of Simulation"; condition "Signal should equal to"
      mask help:
      | The Subsystem checks if the incoming signal (i.e. Overall Verdict, single Requirement Local Verdict, or SUT Outputs) has an expected value at the end of simulation of a previously specified testcase.
      | ____________________________________________________________________
      | 'Check @ End of Simulation' gets the simulation stop time from the window in Simulink.
      | 'Signal should equal to:' is used for giving the condition for the value of signal (i.e.):
      | 2 = none
      | 1 = pass
      | 0 = fail
      | X = anyNumber
      | The subsystem outputs 1 if the condition is fullfilled.
      mask init:
      | % p=get_param(gcb, 'PortHandles');
      | % l=get_param(p.Inport, 'Line'); 
      | % Inp=get_param(p.Inport, 'Name');
      | % set_param(Inp, 'Name', get_param(l, 'Name'));
      mask CallbackString:
      | block = gcb;
      | TCtblock = get_param(get_param(block, 'Parent'), 'Parent');
      | currentStopTime = get_param(TCtblock, 'StopTime');|

== system MIL_Test/Test Data/Feature generation/Generate  feature variants ==
  TestDataVariants Sequence : Stateflow chart

== system MIL_Test/Test Data/Feature generation/Generate  limited decrease ==
  Repeating Sequence : simulink/Sources/Repeating Sequence  SystemSampleTime=-1  rep_seq_t=[0 2]  rep_seq_y=[X0 XF]
  Out1 : Outport
  wires:
  Repeating Sequence/1 -> Out1/1

== system MIL_Test/Test Data/Feature generation/Generate  limited decrease  with slope ==
  Clock : Clock
      settings: Decimation=10
  Constant : Constant  Value=start
  Constant1 : Constant  Value=X0
  Constant2 : Constant  Value=XF
  Constant3 : Constant  Value=XF
  Output : Sum  Inputs=|++  SaturateOnIntegerOverflow=on  InputSameDT=on
  Output1 : Sum  Inputs=|+-+  SaturateOnIntegerOverflow=on  InputSameDT=on
  Output2 : Sum  Inputs=|+-+  SaturateOnIntegerOverflow=on  InputSameDT=on
  Product : Product  SaturateOnIntegerOverflow=on  InputSameDT=on
  RO : RelationalOperator  Operator=<  LogicOutDataTypeMode=Boolean
  RO1 : RelationalOperator  Operator=<  LogicOutDataTypeMode=Boolean
  Step : Step  Time=start  After=slope  SampleTime=0
  Sum : Sum  Inputs=|+-  SaturateOnIntegerOverflow=on  InputSameDT=on
  Switch : Switch  Criteria=u2 > Threshold
  Switch1 : Switch  Criteria=u2 > Threshold
  Out1 : Outport
  wires:
  Clock/1 -> Sum/1
  Constant/1 -> Sum/2
  Sum/1 -> Product/2
  Output/1 -> Output1/1, RO/1, Switch/3
  Constant1/1 -> Output/2, Output1/3, Output2/3
  Product/1 -> Output/1
  Step/1 -> Product/1
  Constant2/1 -> RO/2, Output1/2
  RO/1 -> Switch/2
  Output1/1 -> Switch/1
  Switch/1 -> Switch1/3, Output2/1, RO1/1
  Constant3/1 -> RO1/2, Output2/2
  RO1/1 -> Switch1/2
  Output2/1 -> Switch1/1
  Switch1/1 -> Out1/1

== system MIL_Test/Test Data/Feature generation/Generate  limited increase ==
  Repeating Sequence : simulink/Sources/Repeating Sequence  SystemSampleTime=-1  rep_seq_t=[0 2]  rep_seq_y=[X0 XF]
  Out1 : Outport
  wires:
  Repeating Sequence/1 -> Out1/1

== system MIL_Test/Test Data/Feature generation/Generate  limited increase  with slope ==
  Clock : Clock
      settings: Decimation=10
  Constant : Constant  Value=start
  Constant1 : Constant  Value=X0
  Constant2 : Constant  Value=XF
  Output : Sum  Inputs=|++  SaturateOnIntegerOverflow=on  InputSameDT=on
  Output1 : Sum  Inputs=|+-+  SaturateOnIntegerOverflow=on  InputSameDT=on
  Output2 : Sum  Inputs=|+-+  SaturateOnIntegerOverflow=on  InputSameDT=on
  Output3 : Sum  Inputs=|+-+  SaturateOnIntegerOverflow=on  InputSameDT=on
  Product : Product  SaturateOnIntegerOverflow=on  InputSameDT=on
  RO : RelationalOperator  Operator=>  LogicOutDataTypeMode=Boolean
  RO1 : RelationalOperator  Operator=>  LogicOutDataTypeMode=Boolean
  RO2 : RelationalOperator  Operator=>  LogicOutDataTypeMode=Boolean
  Step : Step  Time=start  After=slope  SampleTime=0
  Sum : Sum  Inputs=|+-  SaturateOnIntegerOverflow=on  InputSameDT=on
  Switch : Switch  Criteria=u2 > Threshold
  Switch1 : Switch  Criteria=u2 > Threshold
  Switch2 : Switch  Criteria=u2 > Threshold
  Out1 : Outport
  wires:
  Step/1 -> Product/1
  Product/1 -> Output/1
  Constant1/1 -> Output/2, Output1/3, Output2/3, Output3/3
  Output/1 -> Output1/1, RO/1, Switch/3  "U(k)"
  Sum/1 -> Product/2
  Constant/1 -> Sum/2
  Clock/1 -> Sum/1
  Constant2/1 -> RO/2, Output1/2, RO1/2, Output2/2, RO2/2, Output3/2
  Switch/1 -> Switch1/3, RO1/1, Output2/1
  Output1/1 -> Switch/1
  RO/1 -> Switch/2
  RO1/1 -> Switch1/2
  Output2/1 -> Switch1/1
  Switch1/1 -> Switch2/3, RO2/1, Output3/1
  Switch2/1 -> Out1/1
  RO2/1 -> Switch2/2
  Output3/1 -> Switch2/1

== system MIL_Test/Test Data/Feature generation/Generate  local maximum  @ given time  ==
  Repeating Sequence : simulink/Sources/Repeating Sequence  SystemSampleTime=-1  rep_seq_t=[0 maxt maxt+1]  rep_seq_y=[X0 XF-X0+20 X0]
  Maximum : Outport
  wires:
  Repeating Sequence/1 -> Maximum/1

== system MIL_Test/Test Data/Feature generation/Generate  local maximum  with given slope ==
  Clock : Clock
      settings: DisableCoverage=on  Decimation=10
  Limited Ramp Increasing : Subsystem
  Limited Ramp  Decreasing1 : Subsystem
  Logical Operator : Logic  AllPortsSameDT=off  OutDataTypeMode=Boolean
  NoStartOfSignal1 : Switch  Criteria=u2 > Threshold
  RO : RelationalOperator  Operator=<  LogicOutDataTypeMode=Boolean
  Sum : Sum  Inputs=|++
  XO : Constant  DisableCoverage=on  Value=X0
  XO1 : Constant  DisableCoverage=on  Value=X0
  startTimeOfMax : Constant  DisableCoverage=on  Value=maxt
  stopped : RelationalOperator  Operator=>  LogicOutDataTypeMode=Boolean
  Maximum : Outport
  wires:
  Logical Operator/1 -> NoStartOfSignal1/2
  stopped/1 -> Logical Operator/2
  RO/1 -> Logical Operator/1
  XO1/1 -> RO/2
  startTimeOfMax/1 -> stopped/2
  Clock/1 -> stopped/1
  Limited Ramp Increasing/2(MaxValue2) -> Limited Ramp  Decreasing1/1(InitialValue)
  Limited Ramp Increasing/1(Out2) -> Sum/1
  NoStartOfSignal1/1 -> Maximum/1
  XO/1 -> NoStartOfSignal1/1
  Sum/1 -> NoStartOfSignal1/3
  Limited Ramp  Decreasing1/1(Out1) -> RO/1, Sum/2

== system MIL_Test/Test Data/Feature generation/Generate  local maximum = maxvalue  @ given time ==
  Repeating Sequence : simulink/Sources/Repeating Sequence  SystemSampleTime=-1  rep_seq_t=[0 maxt maxt+1]  rep_seq_y=[X0 maxv X0]
  Maximum : Outport
  wires:
  Repeating Sequence/1 -> Maximum/1

== system MIL_Test/Test Data/Feature generation/Generate any step response  characteristics ==
  Plant : TransferFcn  Numerator=[10]  Denominator=[1 1 10]
  Scope : Scope  NumInputPorts=5
      settings: YMin=-5~-5~-5~-5~-5  YMax=5~5~5~5~5  MaxDataPoints=1115000
  Step1 : Step  Time=2  SampleTime=0
  Sum : Sum  Inputs=|+-
  Step response : Outport
  wires:
  Sum/1 -> Plant/1
  Step1/1 -> Sum/1  "Step"
  Plant/1 -> Step response/1, Sum/2, Scope/1  "Step response"

== system MIL_Test/Test Data/Feature generation/Generate complete step ==
  InOut Bus : Inport
  Bus Selector : BusSelector  OutputSignals=signal2.T
  Clock1 : Clock
      settings: Decimation=10
  Data Store : DataStoreMemory  StartFcn=triggerTime=triggerTime +50;  DataStoreName=triggerTime  InitialValue=0
  Generate step : Step  InitFcn=triggerTime=0;  StartFcn=triggerTime=triggerTime+50;  Time=150  Before=100  After=40  SampleTime=0
  Generate step1 : Step  Time=100  Before=80  After=100  SampleTime=0
  Hold Time : Subsystem  TreatAsAtomicUnit=on
  Hold Value : Subsystem  TreatAsAtomicUnit=on
  Memory : Memory
  Relational Operator : RelationalOperator  Operator===  LogicOutDataTypeMode=Boolean
  Switch : Switch  Criteria=u2 > Threshold
  triggered : Constant
  v_Des : Outport
  wires:
  Bus Selector/1 -> Memory/1  "<T>"
  Memory/1 -> Relational Operator/1
  Clock1/1 -> Hold Time/1(Clock)
  Hold Value/1(v_Des) -> Switch/2
  Switch/1 -> v_Des/1
  Generate step1/1 -> Switch/3
  Generate step/1 -> Switch/1
  Relational Operator/1 -> Hold Time/Enable, Hold Value/Enable, Hold Value/1(In1)
  triggered/1 -> Relational Operator/2
  InOut Bus/1 -> Bus Selector/1

== system MIL_Test/Test Data/Feature generation/Generate linear relation ==
  Clock : Clock
      settings: DisableCoverage=on  Decimation=10
  Product : Product  DisableCoverage=on  SaturateOnIntegerOverflow=on  InputSameDT=on
  Step : Step  DisableCoverage=on  Time=0  After=c  SampleTime=0
  Out1 : Outport
  wires:
  Clock/1 -> Product/2
  Product/1 -> Out1/1
  Step/1 -> Product/1

== system MIL_Test/Test Data/Feature generation/Generate min to date ==
  Sine Wave : Sin  SampleTime=0
  Step1 : Step  Time=2  SampleTime=0
  Step2 : Step  Time=5  Before=up  After=low  SampleTime=0
  Sum : Sum  Inputs=|+++
  Min to date : Outport
  wires:
  Step1/1 -> Sum/1  "Step"
  Sum/1 -> Min to date/1
  Step2/1 -> Sum/2
  Sine Wave/1 -> Sum/3

== system MIL_Test/Test Data/Feature generation/Generate peaks ==
  Repeating Sequence : simulink/Sources/Repeating Sequence  SystemSampleTime=-1  rep_seq_t=[0 1/freq]  rep_seq_y=[Sens -Sens]
  Peak : Outport
  wires:
  Repeating Sequence/1 -> Peak/1

== system MIL_Test/Test Data/Feature generation/Generate signal  crossing a given value  @ given time ==
  Step : Step  Time=time  Before=up-low+1  After=val  SampleTime=0
  Feature : Outport
  wires:
  Step/1 -> Feature/1

== system MIL_Test/Test Data/Feature generation/Generate signal which  starts to be constant @ time ==
  Clock1 : Clock
      settings: Decimation=10
  Constant : Constant  Value=const
  Relational Operator : RelationalOperator  LogicOutDataTypeMode=Boolean
  Sine Wave : Sin  SampleTime=0
  Switch1 : Switch  Criteria=u2 > Threshold
  start time : Constant  Value=ST
  Feature : Outport
  wires:
  Clock1/1 -> Relational Operator/1
  start time/1 -> Relational Operator/2
  Relational Operator/1 -> Switch1/2
  Constant/1 -> Switch1/1
  Sine Wave/1 -> Switch1/3
  Switch1/1 -> Feature/1

== system MIL_Test/Test Data/Signal comparison/Bound Precond ==
  Signal : Inport
  Reference : Inport  Port=2
  RelOp : RelationalOperator  LogicOutDataTypeMode=Specify via dialog
  Activate : Outport
  wires:
  Reference/1 -> RelOp/2
  RelOp/1 -> Activate/1
  Signal/1 -> RelOp/1
